simulink model "FlexibleJoint_model"  (R2021a)
settings: Solver=VariableStepAuto  StartTime=0.0  StopTime=20  RelTol=1e-3
undefined symbols (not defined in the file): Base_model_2
libraries: cstblocks x3, simulink x1
settings Model: Creator=andre  LastModifiedBy=andre

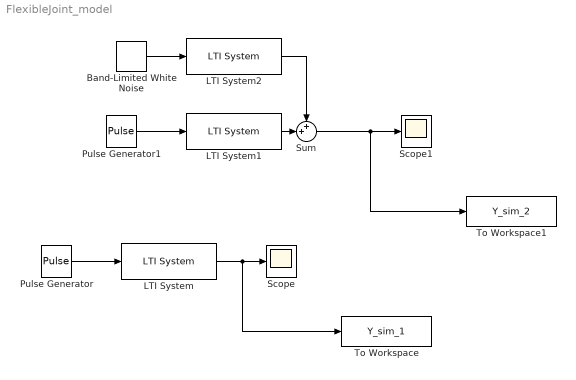
== system FlexibleJoint_model ==
  Band-Limited White Noise : simulink/Sources/Band-Limited White Noise  Cov=[0.1]  Ts=0.002  seed=[23341]
  LTI System : cstblocks/LTI System  sys=Base_model_1  IC=[]
  LTI System1 : cstblocks/LTI System  sys=Base_model_2  IC=[]
  LTI System2 : cstblocks/LTI System  sys=tf(Base_model_2, 'noise')  IC=[]
  Pulse Generator : DiscretePulseGenerator  PulseType=Time based  Amplitude=5  Period=5  PulseWidth=5
  Pulse Generator1 : DiscretePulseGenerator  PulseType=Time based  Amplitude=5  Period=5  PulseWidth=5
  Scope : Scope
  Scope1 : Scope
  Sum : Sum  Inputs=++|
  To Workspace : ToWorkspace  VariableName=Y_sim_1  SaveFormat=Timeseries  SampleTime=0.002
  To Workspace1 : ToWorkspace  VariableName=Y_sim_2  SaveFormat=Timeseries  SampleTime=0.002
  wires:
  Sum/1 -> To Workspace1/1, Scope1/1
  Band-Limited White Noise/1 -> LTI System2/1
  LTI System2/1 -> Sum/1
  LTI System1/1 -> Sum/2
  Pulse Generator1/1 -> LTI System1/1
  Pulse Generator/1 -> LTI System/1
  LTI System/1 -> To Workspace/1, Scope/1
